simulink model "heat_exchanger_exact_linearization"  (R2017b)
settings: Solver=VariableStepAuto  StartTime=0.0  StopTime=10000  RelTol=1e-3
values from neighbouring files (symbols this model uses):
  Area = n*A_heat_plate    (= 9.8716)    [heat_exchanger_config.m]    (also in linearization.m = 20)
  cp_H2O = 4190    [heat_exchanger_config.m]    (also in linearization.m)
  cp_wort = 4062    [heat_exchanger_config.m]    (also in linearization.m = 4000)
  Kr = inv(D-(C-D*LQR_gain)*inv(A-B*LQR_gain))    [heat_exchanger_config.m]
  m_H2O = m_wort    (= 10)    [heat_exchanger_config.m]    (also in linearization.m = 1)
  m_wort = 10    [heat_exchanger_config.m]    (also in linearization.m = 1)
  Reference = [20 70]    [heat_exchanger_config.m]    (also in linearization.m = [25 16])
  T_H2O_in = 5    [heat_exchanger_config.m]    (also in linearization.m = 10)
  T_wort_in = 95    [heat_exchanger_config.m]    (also in linearization.m = 70)
  U = (m_dot_h_data*cp_wort*(T_wort_in-T_wort_out)*log(Delta_T2/Delta_T1))/     (Area*(Delta_T2-Delta_T1))    [heat_exchanger_config.m]    (also in linearization.m = 1000)
undefined symbols (not defined in the file or in its folder): LQR_gain
settings Model: Creator=Alexander  LastModifiedBy=Alexander

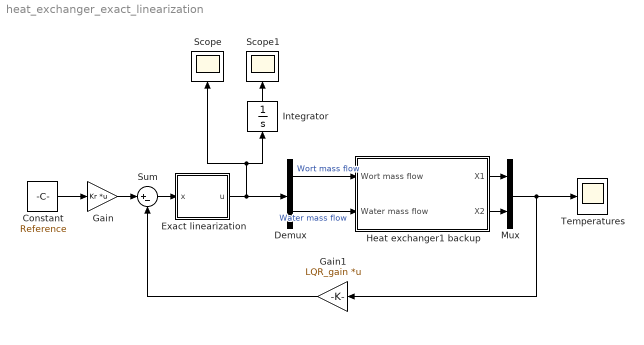
== system heat_exchanger_exact_linearization ==
  Constant : Constant  Value=Reference
  Demux : Demux  Outputs=2
  Exact linearization : Subsystem
  Gain : Gain  Gain=Kr  Multiplication=Matrix(K*u) (u vector)
  Gain1 : Gain  Gain=LQR_gain  Multiplication=Matrix(K*u) (u vector)
  Heat exchanger1 backup : Subsystem
  Integrator : Integrator
  Mux : Mux  Inputs=2
  Scope : Scope
  Scope1 : Scope
  Sum : Sum  Inputs=|+-
  Temperatures : Scope
  wires:
  Demux/2 -> Heat exchanger1 backup/2(Water mass flow)  "Water mass flow"
  Heat exchanger1 backup/2(X2) -> Mux/2
  Heat exchanger1 backup/1(X1) -> Mux/1
  Demux/1 -> Heat exchanger1 backup/1(Wort mass flow)  "Wort mass flow"
  Constant/1 -> Gain/1
  Exact linearization/1(u) -> Demux/1, Integrator/1, Scope/1
  Mux/1 -> Gain1/1, Temperatures/1
  Sum/1 -> Exact linearization/1("x ")
  Gain/1 -> Sum/1
  Gain1/1 -> Sum/2
  Integrator/1 -> Scope1/1

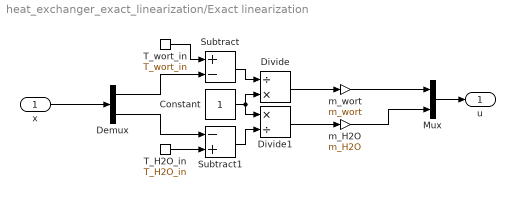
== system heat_exchanger_exact_linearization/Exact linearization ==
  "x " : Inport
  Constant : Constant
  Demux : Demux  Outputs=2
  Divide : Product  Inputs=/*
  Divide1 : Product  Inputs=*/
  Mux : Mux  Inputs=2
  Subtract : Sum  Inputs=+-
  Subtract1 : Sum  Inputs=-+
  T_H2O_in : Constant  Value=T_H2O_in
  T_wort_in : Constant  Value=T_wort_in
  m_H2O : Gain  Gain=m_H2O
  m_wort : Gain  Gain=m_wort
  u : Outport
  wires:
  "x "/1 -> Demux/1
  Mux/1 -> u/1
  m_wort/1 -> Mux/1
  Divide/1 -> m_wort/1
  Constant/1 -> Divide1/1, Divide/2
  Demux/1 -> Subtract/2
  T_wort_in/1 -> Subtract/1
  Subtract/1 -> Divide/1
  m_H2O/1 -> Mux/2
  Divide1/1 -> m_H2O/1
  Subtract1/1 -> Divide1/2
  Demux/2 -> Subtract1/1
  T_H2O_in/1 -> Subtract1/2

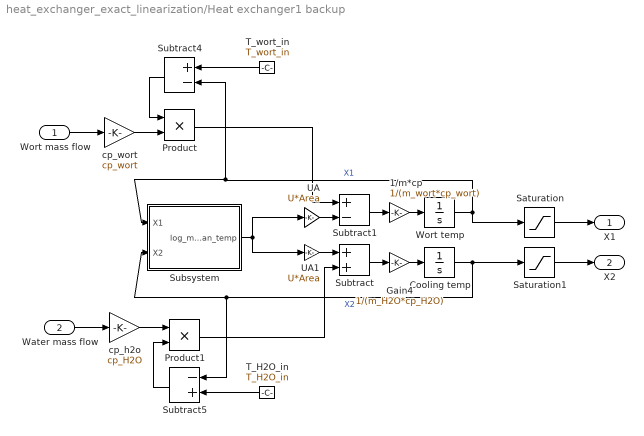
== system heat_exchanger_exact_linearization/Heat exchanger1 backup ==
  Wort mass flow : Inport
  Water mass flow : Inport  Port=2
  "1/m*cp " : Gain  Gain=1/(m_wort*cp_wort)
  Cooling temp : Integrator  InitialCondition=T_H2O_in-0.1
  Gain4 : Gain  Gain=1/(m_H2O*cp_H2O)
  Product : Product
  Product1 : Product
  Saturation : Saturate  UpperLimit=T_wort_in  LowerLimit=T_H2O_in
  Saturation1 : Saturate  UpperLimit=T_wort_in  LowerLimit=T_H2O_in
  Subsystem : Subsystem
  Subtract : Sum
  Subtract1 : Sum  Inputs=+-
  Subtract4 : Sum  Inputs=+-
  Subtract5 : Sum  Inputs=-+
  T_H2O_in : Constant  Value=T_H2O_in
  T_wort_in : Constant  Value=T_wort_in
  UA : Gain  Gain=U*Area
  "UA1 " : Gain  Gain=U*Area
  Wort temp : Integrator  InitialCondition=T_wort_in-0.1
  cp_h2o : Gain  Gain=cp_H2O
  cp_wort : Gain  Gain=cp_wort
  X1 : Outport
  X2 : Outport  Port=2
  wires:
  Cooling temp/1 -> Saturation1/1, Subtract5/1, Subsystem/2(X2)  "X2"
  "1/m*cp "/1 -> Wort temp/1
  Wort temp/1 -> Saturation/1, Subsystem/1("X1 "), Subtract4/2  "X1"
  UA/1 -> Subtract1/2
  Subtract1/1 -> "1/m*cp "/1
  Gain4/1 -> Cooling temp/1
  "UA1 "/1 -> Subtract/1
  Subtract/1 -> Gain4/1
  T_wort_in/1 -> Subtract4/1
  Subtract5/1 -> Product1/2
  Product/1 -> Subtract1/1
  T_H2O_in/1 -> Subtract5/2
  Subtract4/1 -> Product/1
  Water mass flow/1 -> cp_h2o/1
  Wort mass flow/1 -> cp_wort/1
  Product1/1 -> Subtract/2
  cp_h2o/1 -> Product1/1
  cp_wort/1 -> Product/2
  Subsystem/1(log_mean_temp) -> UA/1, "UA1 "/1
  Saturation/1 -> X1/1
  Saturation1/1 -> X2/1

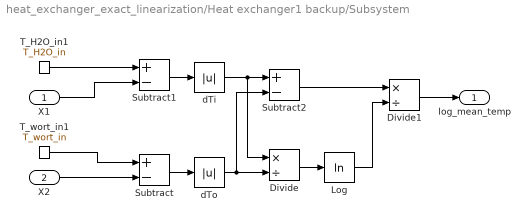
== system heat_exchanger_exact_linearization/Heat exchanger1 backup/Subsystem ==
  "X1 " : Inport
  X2 : Inport  Port=2
  Divide : Product  Inputs=*/
  Divide1 : Product  Inputs=*/
  Log : Math  Operator=log  SaturateOnIntegerOverflow=on
  Subtract : Sum  Inputs=+-
  Subtract1 : Sum  Inputs=+-
  Subtract2 : Sum  Inputs=+-
  T_H2O_in1 : Constant  Value=T_H2O_in
  T_wort_in1 : Constant  Value=T_wort_in
  dTi : Abs
  dTo : Abs
  log_mean_temp : Outport
  wires:
  Subtract/1 -> dTo/1
  T_wort_in1/1 -> Subtract/1
  X2/1 -> Subtract/2
  Subtract1/1 -> dTi/1
  "X1 "/1 -> Subtract1/2
  T_H2O_in1/1 -> Subtract1/1
  dTo/1 -> Subtract2/2, Divide/2
  dTi/1 -> Subtract2/1, Divide/1
  Divide/1 -> Log/1
  Log/1 -> Divide1/2
  Divide1/1 -> log_mean_temp/1
  Subtract2/1 -> Divide1/1
